simulink library "sandbox_lib"  (Simulink 8.6)
settings: Solver=VariableStepAuto  StartTime=0.0  StopTime=10.0  RelTol=1e-3
settings Model: Creator=j.bolting  LastModifiedBy=j.bolting

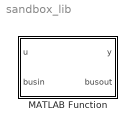
== system sandbox_lib ==
  MATLAB Function : MATLAB Function  TreatAsAtomicUnit=on

== matlab function MATLAB Function ==
  data: u input double; y output double; busin input Bus: VortexBus size=1; busout output Bus: VortexBus size=1; Sig data_store_memory double
function [y, busout] = fcn(u, busin)
%#codegen
global Sig;

test = zeros(3);
test = ffb_quat2dcm([1 0 0 0]);

id = 1;
busout = busin;
busout.alpha_rad(id) = 0.123;
busout.p_NED_m(:, id) = [1 2 3]';
busout.v_NED_mps(:, id) = [1 2 3]';

Sig(10).alpha = Sig(10).alpha + 1;
y = Sig(10).alpha;

end
